simulink model "QPSK_Lecture11"  (R2018b)
settings: Solver=VariableStepAuto  StartTime=0.0  StopTime=inf  RelTol=1e-3
InitFcn:
  | QPSK_ini
undefined symbols (not defined in the file or in its folder): rolloff_factor
libraries: commutil2 x2, commdigbbndpm3 x2, commfilt2 x2, commrandsrc3 x1, commchan3 x1, dspsigops x1
settings Model: Creator=Arthur  LastModifiedBy=Arthur
settings SFSimCC: SimUseLocalCustomCode=off
settings RTWCC: RTWUseLocalCustomCode=off
settings CodeAppCC: StateflowObjectComments=on

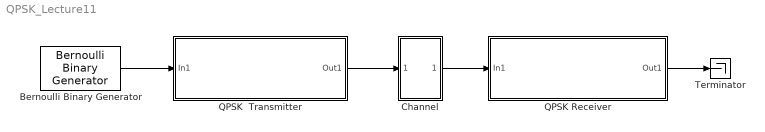
== system QPSK_Lecture11 ==
  Bernoulli Binary Generator : commrandsrc3/Bernoulli Binary Generator  ProbabilityOfZero=0.5  SeedSource=Auto  Seed=0  SampleTime=1  SamplesPerFrame=512  OutputDataType=double  SimulateUsing=Interpreted execution
      settings: SourceProductName=Communications Toolbox
  Channel : Subsystem
  QPSK  Transmitter : Subsystem
  QPSK Receiver : Subsystem
  Terminator : Terminator
  wires:
  Bernoulli Binary Generator/1 -> QPSK  Transmitter/1(In1)
  QPSK  Transmitter/1(Out1) -> Channel/1(In1)
  Channel/1(Out1) -> QPSK Receiver/1(In1)
  QPSK Receiver/1(Out1) -> Terminator/1

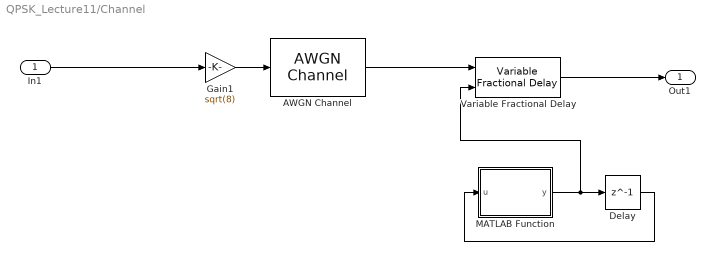
== system QPSK_Lecture11/Channel ==
  In1 : Inport
  AWGN Channel : commchan3/AWGN Channel  InputProcessing=Columns as channels (frame based)  seed=67  noiseMode="Signal to noise ratio  (Eb/No)"  EbNodB=20  EsNodB=10  SNRdB=10  bitsPerSym=2  Ps=1  Tsym=1  variance=1
      settings: SourceProductName=Communications Toolbox
  Delay : Delay  DelayLength=1
  Gain1 : Gain  Gain=sqrt(8)
  MATLAB Function : MATLAB Function  TreatAsAtomicUnit=on
  Variable Fractional Delay : dspsigops/Variable Fractional Delay  mode=OBSOLETE  modeActive=Linear  L=4  FarrowL=4  R=10  alpha=1  dmax=30000  InputProcessing=Columns as channels (frame based)  ic=0  noDFT=off  fallbackFIR=Clip to the minimum value necessary for centered kernel  fallbackFarrow=Clip to the minimum value necessary for centered kernel  roundingMode=Zero  overflowMode=off
      settings: SourceProductName=DSP System Toolbox  SourceProductBaseCode=DS
  Out1 : Outport
  wires:
  Gain1/1 -> AWGN Channel/1
  AWGN Channel/1 -> Variable Fractional Delay/1
  Variable Fractional Delay/1 -> Out1/1
  Delay/1 -> MATLAB Function/1(u)
  MATLAB Function/1(y) -> Variable Fractional Delay/2, Delay/1
  In1/1 -> Gain1/1

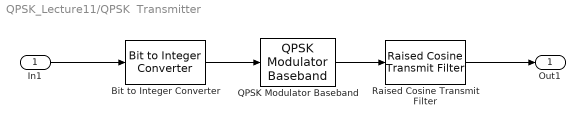
== system QPSK_Lecture11/QPSK  Transmitter ==
  In1 : Inport
  Bit to Integer Converter : commutil2/Bit to Integer Converter  nbits=2  bitOrder=MSB first  signedOutputValues=Unsigned  outDtype=Inherit via internal rule  outDtypeSigned=Inherit via internal rule
      settings: SourceProductName=Communications Toolbox
  QPSK Modulator Baseband : commdigbbndpm3/QPSK Modulator Baseband  InType=Integer  Enc=Gray  Ph=pi/4  outDtype=double  outWordLen=16  outUDDataType=sfix(16)  outFracLenMode=Best precision  outFracLen=15  outDataTypeStr=double  outLastDataTypeStr=double
      settings: SourceProductName=Communications Toolbox
  Raised Cosine Transmit Filter : commfilt2/Raised Cosine Transmit Filter  filtType=Square root  R=rolloff_factor  filtSpan=10  N=4  filterGain=1  InputProcessing=Columns as channels (frame based)  RateOptions=Enforce single-rate processing  framing=Mute  checkCoeff=off  variableName=rcTxFilt  checkGain=Normalized  sampMode=Mute  saveAsFlag=0  currentFiltSpan=10  D=5  launchFVT=on  roundingMode=Floor  overflowMode=off  coeffDataTypeStr=Inherit: Same word length as input  coeffMin=[]  coeffMax=[]  coeffLastDataTypeStr=Inherit: Same word length as input  outputDataTypeStr=Inherit: Same as accumulator  outputMin=[]  outputMax=[]  outputLastDataTypeStr=Inherit: Same as accumulator
      settings: SourceProductName=Communications Toolbox
  Out1 : Outport
  wires:
  In1/1 -> Bit to Integer Converter/1
  Bit to Integer Converter/1 -> QPSK Modulator Baseband/1
  QPSK Modulator Baseband/1 -> Raised Cosine Transmit Filter/1
  Raised Cosine Transmit Filter/1 -> Out1/1

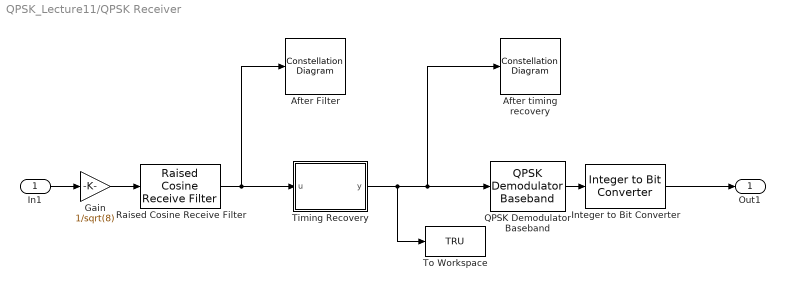
== system QPSK_Lecture11/QPSK Receiver ==
  In1 : Inport
  After Filter : ConstellationDiagram
  "After timing recovery " : ConstellationDiagram
  Gain : Gain  Gain=1/sqrt(8)
  Integer to Bit Converter : commutil2/Integer to Bit Converter  nbits=2  signedInputValues=Unsigned  bitOrder=MSB first  outDtype=Inherit via internal rule
      settings: SourceProductName=Communications Toolbox
  QPSK Demodulator Baseband : commdigbbndpm3/QPSK Demodulator Baseband  OutType=Integer  DecType=Hard decision  VarSource=Dialog  Variance=1  Dec=Gray  Ph=pi/4  outDtype1=Inherit via internal rule  outDtype2=Inherit via internal rule  derotateFactorWordLen=16  derotateFactorDataTypeStr=Inherit: Same word length as input  derotateFactorLastDataTypeStr=Inherit: Same word length as input
      settings: SourceProductName=Communications Toolbox
  Raised Cosine Receive Filter : commfilt2/Raised Cosine Receive Filter  filtType=Square root  R=0.2  filtSpan=10  N=4  downFactor=1  downOffset=0  filterGain=1  InputProcessing=Columns as channels (frame based)  RateOptions=Enforce single-rate processing  framing=Mute  checkCoeff=off  variableName=rcRxFilt  currentFiltSpan=10  D=5  inputOffset=0  sampMode=Mute  saveAsFlag=0  rateMode=Downsampling  checkGain=Normalized  launchFVT=on  roundingMode=Floor  overflowMode=off  coeffDataTypeStr=Inherit: Same word length as input  coeffMin=[]  coeffMax=[]  coeffLastDataTypeStr=Inherit: Same word length as input  accumDataTypeStr=Inherit: Same as product output  accumLastDataTypeStr=Inherit: Same as product output  outputDataTypeStr=Inherit: Same as accumulator  outputMin=[]  outputMax=[]  outputLastDataTypeStr=Inherit: Same as accumulator
      settings: SourceProductName=Communications Toolbox
  Timing Recovery : MATLAB Function  TreatAsAtomicUnit=on
  To Workspace : ToWorkspace  VariableName=TRU  SampleTime=-1
  Out1 : Outport
  wires:
  In1/1 -> Gain/1
  Raised Cosine Receive Filter/1 -> Timing Recovery/1(u), After Filter/1
  QPSK Demodulator Baseband/1 -> Integer to Bit Converter/1
  Gain/1 -> Raised Cosine Receive Filter/1
  Integer to Bit Converter/1 -> Out1/1
  Timing Recovery/1(y) -> To Workspace/1, QPSK Demodulator Baseband/1, "After timing recovery "/1

== matlab function QPSK_Lecture11/QPSK Receiver/Timing Recovery ==
  data: u input; y output
function y = fcn(u)

persistent yva yvs

if isempty(yva)
    yva = zeros(4,1);
    yvs = zeros(4,1);
end

d = length(u);
y = complex(zeros(d/4,1));
rho = 0.08;
for m=4:4:d
    yva(1,1) = (1-rho)*yva(1,1)+rho*abs(u(m-3));
    yva(2,1) = (1-rho)*yva(2,1)+rho*abs(u(m-2));
    yva(3,1) = (1-rho)*yva(3,1)+rho*abs(u(m-1));
    yva(4,1) = (1-rho)*yva(4,1)+rho*abs(u(m));
    yvs(1,1) = (1-rho)*yvs(1,1)+rho*abs(abs(u(m-3)-yva(1,1)));
    yvs(2,1) = (1-rho)*yvs(2,1)+rho*abs(abs(u(m-2)-yva(2,1)));
    yvs(3,1) = (1-rho)*yvs(3,1)+rho*abs(abs(u(m-1)-yva(3,1)));
    yvs(4,1) = (1-rho)*yvs(4,1)+rho*abs(abs(u(m)-yva(4,1)));
end
[~,index] = min([yvs(1) yvs(2) yvs(3) yvs(4)]);

== matlab function QPSK_Lecture11/Channel/MATLAB Function ==
  data: u input; y output
function y = fcn(u)

y = u + 0.001;
